simulink model "kinematic_controller_system"  (R2013a)
settings: Solver=ode45  StartTime=0.0  StopTime=100  FixedStep=0.1  RelTol=1e-3
libraries: simulink x4, DiffSteer_model x2, Controllers x2
settings Model: Creator=Felipe  LastModifiedBy=Felipe
settings DebuggingCC: SolverPrmCheckMsg=none

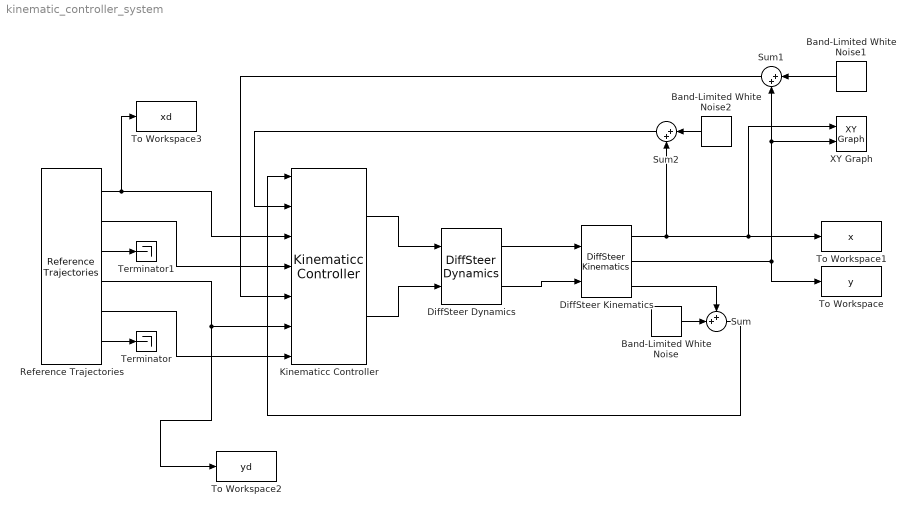
== system kinematic_controller_system ==
  Band-Limited White Noise : simulink/Sources/Band-Limited White Noise  Cov=[0]  Ts=0.1  seed=[23341]
  Band-Limited White Noise1 : simulink/Sources/Band-Limited White Noise  Cov=[0]  Ts=0.1  seed=[03341]
  Band-Limited White Noise2 : simulink/Sources/Band-Limited White Noise  Cov=[0]  Ts=0.1  seed=[20341]
  DiffSteer Dynamics : DiffSteer_model/DiffSteer Dynamics  umax=0.75  wmax=1.745  dumax=0.3  dwmax=1.745  param=[0.2604 0.2509 -0.000499 0.9965 0.00263 1.0768]
  DiffSteer Kinematics : DiffSteer_model/DiffSteer Kinematics  x0=[-0.5, -0.5, pi]  a=0.2  umax=0.75  wmax=1.745  dumax=0.3  dwmax=1.745
  Kinematicc Controller : Controllers/Kinematicc Controller  kx=10  ky=10  lx=10  ly=10  a=0.2
  Reference Trajectories : Controllers/Reference Trajectories  trajectory_type=2  wf=0.25  raio_ref_1=1  delta_raio=-0.1  t_delta_raio=60  xd=[1, -2.5]
  Sum : Sum  Inputs=++|
  Sum1 : Sum  Inputs=|++
  Sum2 : Sum  Inputs=|++
  Terminator : Terminator
  Terminator1 : Terminator
  To Workspace : ToWorkspace  VariableName=y  SampleTime=-1
  To Workspace1 : ToWorkspace  VariableName=x  SampleTime=-1
  To Workspace2 : ToWorkspace  VariableName=yd  SampleTime=-1
  To Workspace3 : ToWorkspace  VariableName=xd  SampleTime=-1
  XY Graph : simulink/Sinks/XY Graph  xmin=-2  xmax=2  ymin=-3  ymax=1  st=-1
  wires:
  Reference Trajectories/1 -> Kinematicc Controller/3, To Workspace3/1
  Reference Trajectories/2 -> Kinematicc Controller/4
  Reference Trajectories/4 -> To Workspace2/1, Kinematicc Controller/6
  Reference Trajectories/5 -> Kinematicc Controller/7
  DiffSteer Kinematics/1 -> Sum2/2, XY Graph/1, To Workspace1/1
  DiffSteer Kinematics/2 -> XY Graph/2, Sum1/2, To Workspace/1
  Kinematicc Controller/1 -> DiffSteer Dynamics/1
  Kinematicc Controller/2 -> DiffSteer Dynamics/2
  DiffSteer Dynamics/1 -> DiffSteer Kinematics/1
  DiffSteer Dynamics/2 -> DiffSteer Kinematics/2
  Reference Trajectories/3 -> Terminator1/1
  Reference Trajectories/6 -> Terminator/1
  DiffSteer Kinematics/3 -> Sum/1
  Band-Limited White Noise/1 -> Sum/2
  Sum/1 -> Kinematicc Controller/1
  Band-Limited White Noise1/1 -> Sum1/1
  Sum1/1 -> Kinematicc Controller/5
  Band-Limited White Noise2/1 -> Sum2/1
  Sum2/1 -> Kinematicc Controller/2
